simulink model "Simulink_drone_BO_facultatif"  (R2025b)
settings: Solver=VariableStepAuto  StartTime=0.0  StopTime=60  RelTol=1e-3
undefined symbols (not defined in the file): bool, controller, dt_realtime, sysBO, x_init
libraries: aerolibanimutils x2, uavsim3dlib x1, sim3dlib x1
settings Model: Creator=guilb  LastModifiedBy=guilb

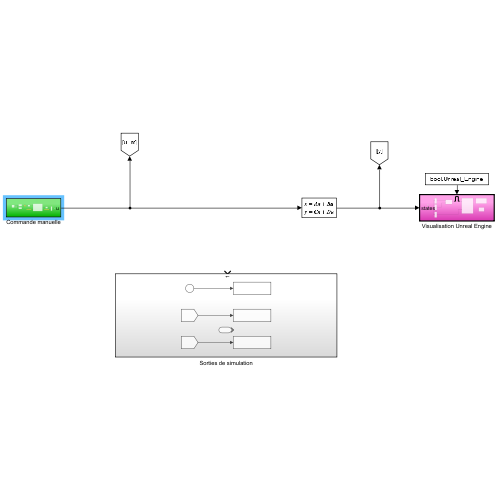
[thumbnail: Simulink's stored preview of the top-level diagram]
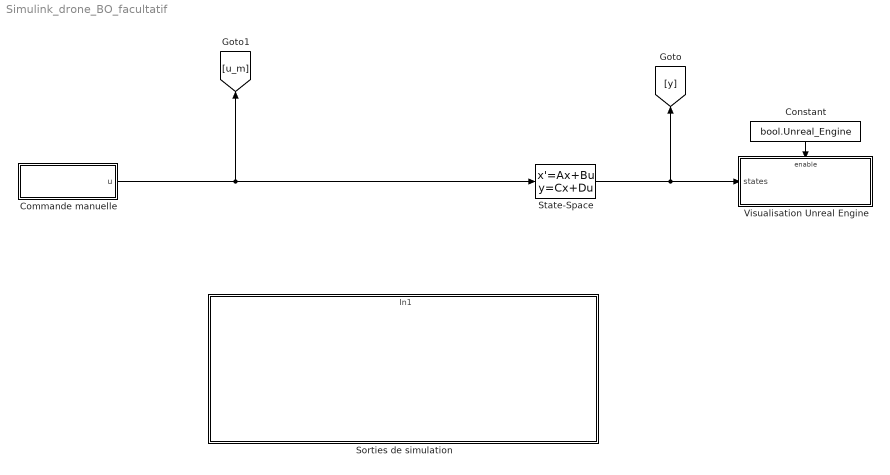
== system Simulink_drone_BO_facultatif ==
  Commande manuelle : Subsystem
  Constant : Constant  Value=bool.Unreal_Engine
  Sorties de simulation : Subsystem
      settings: PortSchema="{\"entries\":[{\"content\":{\"sides\":[{\"content\":{},\"type\":\"ConnectorPlacement.EquallySpacedRectSide\",\"uuid\":\"13ffba7f-bf1d-45b8-ba16-d739f7cf7d65\"},{\"content\":{\"side\":\"RIGHT\"},\"type\":\"ConnectorPlacement.EquallySpacedRectSide\",\"uuid\":\"a06d5891-851d-4d6f-ac4a-718ff50ccabc\"},{\"content\":{\"connectorIds\":[\"In1\"],\"side\":\"TOP\"},\"type\":\"ConnectorPlacement.EquallySpacedRectSide\",\"uuid\":\"896d5570-b42a-4582-b469-16ee5988ede6\"}]},\"type\":\"ConnectorPlacement.EquallySpacedConnector\",\"uuid\":\"8422d13c-e10a-49e8-a54f-6123e5432cb6\"}],\"packageUris\":[\"http://schema.mathworks.com/mf0/Connector/R2020b\"],\"version\":\"1.0\"}"
  State-Space : StateSpace  A=sysBO.A  B=sysBO.B  C=sysBO.C  D=sysBO.D  InitialCondition=x_init
  Visualisation Unreal Engine : Subsystem
  wires:
  Constant/1 -> Visualisation Unreal Engine/Enable
  State-Space/1 -> Visualisation Unreal Engine/1(states), [y]
  Commande manuelle/1(u) -> State-Space/1, [u_m]

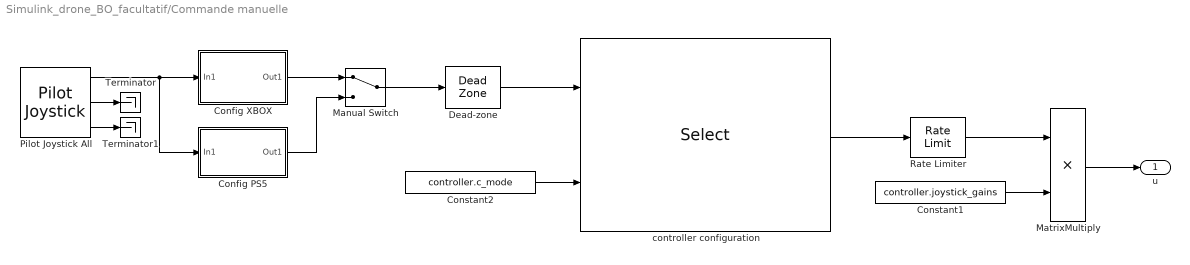
== system Simulink_drone_BO_facultatif/Commande manuelle ==
  Config PS5 : Subsystem
      mask Display: image('controller_ps5.png', [2,2,2,2,100,100]);
  "Config XBOX " : Subsystem
      mask Display: image('controller_xbox.png', [2,2,2,2,100,100]);
  Constant1 : Constant  Value=controller.joystick_gains
  Constant2 : Constant  Value=controller.c_mode
  Dead-zone : DeadZone  LowerValue=-0.2  UpperValue=0.2
  Manual Switch : ManualSwitch
  MatrixMultiply : Product
  Pilot Joystick All : aerolibanimutils/Pilot Joystick  JoystickID=Joystick1  OutputConfiguration=AllOutputs  SampleTime=dt_realtime
      settings: LibrarySourceBlock=aerolibanimutils/Pilot Joystick All
  "Rate Limiter " : RateLimiter  RisingSlewLimit=controller.rate_limits  FallingSlewLimit=-controller.rate_limits
  Terminator : Terminator
  Terminator1 : Terminator
  controller configuration : Selector  InputPortWidth=4  IndexOptions=Index vector (port)  Indices=[2 4 3 1]  OutputSizes=1
      mask Display: image('controller_modes.png');
  u : Outport
  wires:
  controller configuration/1 -> "Rate Limiter "/1
  MatrixMultiply/1 -> u/1
  Constant1/1 -> MatrixMultiply/2
  Constant2/1 -> controller configuration/2
  "Rate Limiter "/1 -> MatrixMultiply/1
  Dead-zone/1 -> controller configuration/1
  Pilot Joystick All/1 -> "Config XBOX "/1(In1), Config PS5/1(In1)
  Manual Switch/1 -> Dead-zone/1
  "Config XBOX "/1(Out1) -> Manual Switch/1
  Config PS5/1(Out1) -> Manual Switch/2
  Pilot Joystick All/2 -> Terminator/1
  Pilot Joystick All/3 -> Terminator1/1

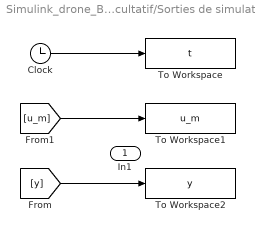
== system Simulink_drone_BO_facultatif/Sorties de simulation ==
  In1 : Inport
  Clock : Clock
  To Workspace : ToWorkspace  VariableName=t  SaveFormat=Timeseries  SampleTime=-1
  To Workspace1 : ToWorkspace  VariableName=u_m  SaveFormat=Timeseries  SampleTime=-1
  To Workspace2 : ToWorkspace  VariableName=y  SaveFormat=Timeseries  SampleTime=-1
  wires:
  Clock/1 -> To Workspace/1
  [y] -> To Workspace2/1
  [u_m] -> To Workspace1/1

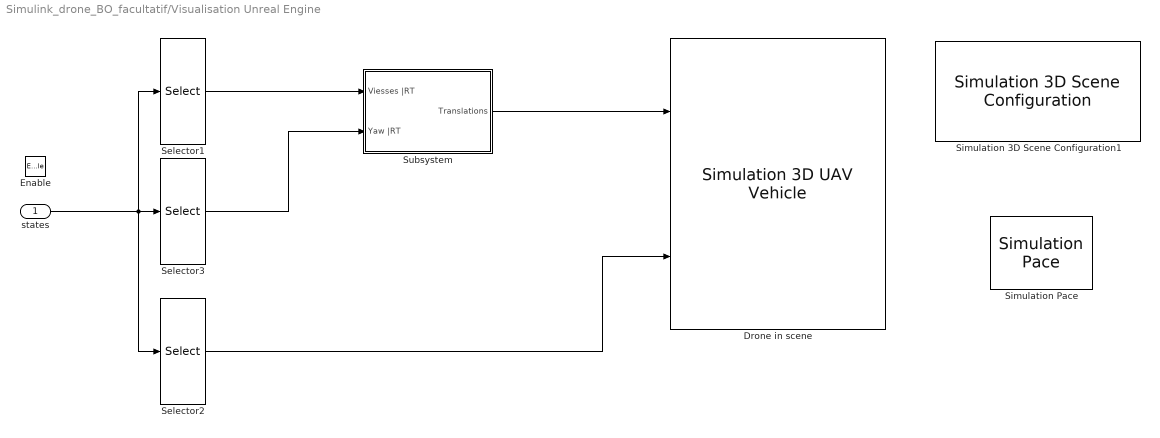
== system Simulink_drone_BO_facultatif/Visualisation Unreal Engine ==
  states : Inport
  Enable : EnablePort
  Drone in scene : uavsim3dlib/Simulation 3D UAV Vehicle  Priority=-1  Mesh=Quadrotor  MeshPath=/MathWorksUAVContent/UAVs/HexaRotorUAV/HexaRotor.HexaRotor  Color=Black  ActorName=SimulinkVehicle1  UseGlobalFrame=off  InitialTranslation=[0 0 0]  InitialRotation=[0 0 0]  InitialTranslationGlobal=[0 0 0]  InitialGeoOrigin=[0 0 0]  InitialRotationGlobal=[0 0 0]  SampleTime=-1  ActorType=SimulinkVehicle  ID=1  aMode=4  ActorTag=SimulinkVehicle1
  Selector1 : Selector  InputPortWidth=12  IndexOptions=Index vector (dialog)  Indices=[2 4 6]  OutputSizes=1
  Selector2 : Selector  InputPortWidth=12  IndexOptions=Index vector (dialog)  Indices=[11 9 7]  OutputSizes=1
  Selector3 : Selector  InputPortWidth=12  IndexOptions=Index vector (dialog)  Indices=11  OutputSizes=1
  Simulation 3D Scene Configuration1 : sim3dlib/Simulation 3D Scene Configuration  Priority=0  ProjectFormat=Default Scenes  SceneDesc=US city block  ProjectName=C:\Program Files\MATLAB\R2025b\toolbox\shared\sim3d_projects\automotive_project_windows\UE\WindowsNoEditor\VehicleSimulation.exe  ScenePath=/Game/Maps/USCityBlock  EnableOpenDRIVE=off  vehTagList={'Custom';'Scene Origin';'SimulinkVehicle1'}  vehTag=SimulinkVehicle1  AttachedCameraRelativeTranslation=[0 0 0]  FreeCameraDefaultInitialTranslation=[-6, 0, 2]  AttachedCameraRelativeRotation=[0 0 0]  FreeCameraDefaultInitialRotation=[0, -15, 0]  ViewpointName=Custom  FreeCameraInitialTranslation=[0, 0, 0]  ViewpointTranslation=[0 0 0]  FreeCameraInitialRotation=[0, 0, 0]  ViewpointRotation=[0 0 0]  OpVisEn=off  Ts=dt_realtime  EnableWindow=on  EnableRemoteAccess=off  EnableWeather=off  SunAzimuth=90  SunAltitude=40.0  EnableGeospatialSun=off  Latitude=0  Longitude=0  Date=2023-01-01  Time=10:30:00  GeoTimeZone=-5.0  SunDaylightSaving=off  wind=1  clouds=10  EnableVolumetricClouds=off  CloudCoverage=0  CloudAltitude=6  fog=0  rain=0  RaindropsEffect=off  SnowDensity=0  EnableGeospatial=off  TilesetSource=Earth terrain  UseTrueOrigin=off  OriginHeight=200  OriginLatitude=40.744652  OriginLongitude=-73.988864  MapStyle=Aerial  AdditionalAssetIDs=[]  UseAdvancedSunSky=off  SolarTime=11  TimeZone=-5  Day=21  Month=9  Year=2022  UseDaylightSavingTime=on  DSTStartDay=10  DSTStartMonth=3  DSTEndDay=3  DSTEndMonth=11  DSTSwitchHour=2  sensorTag=MainCamera1  sensorId=1  sensorName=MainCamera1  mountLoc=Origin  offsetFlag=off  tmountOffset=[0, 0, 0]  rmountOffset=[0, 0, 0]  HorizontalResolution=1280  VerticalResolution=720  HorizontalFOV=60  mountPoint=[0 0 0]  mountOrientation=[0 0 0]  aMode=4  ID=1  GeoTrigger=Inactive  ViewNameList={'Custom'}  ViewTranslationList={'[0 0 0]'}  ViewRotationList={'[0 0 0]'}
      settings: LibrarySourceBlock=uavsim3dlib/Simulation 3D Scene Configuration
  Simulation Pace : aerolibanimutils/Simulation Pace  SimulationPace=1  SleepMode=Auto  OutputPaceError=off  SampleTime=dt_realtime
  Subsystem : Subsystem
  wires:
  states/1 -> Selector1/1, Selector2/1, Selector3/1
  Selector2/1 -> Drone in scene/2
  Selector1/1 -> Subsystem/1(Viesses |RT)
  Selector3/1 -> Subsystem/2("Yaw |RT ")
  Subsystem/1(Translations) -> Drone in scene/1

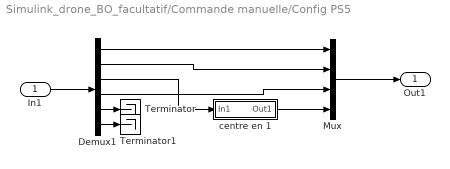
== system Simulink_drone_BO_facultatif/Commande manuelle/Config PS5 ==
  In1 : Inport
  Demux1 : Demux  Outputs=6
  Mux : Mux
  Terminator : Terminator
  Terminator1 : Terminator
  centre en 1 : Subsystem
  Out1 : Outport
  wires:
  Demux1/6 -> Terminator1/1
  Demux1/5 -> Terminator/1
  Demux1/4 -> Mux/3
  In1/1 -> Demux1/1
  Demux1/1 -> Mux/1
  Demux1/2 -> Mux/2
  Mux/1 -> Out1/1
  centre en 1/1(Out1) -> Mux/4
  Demux1/3 -> centre en 1/1(In1)

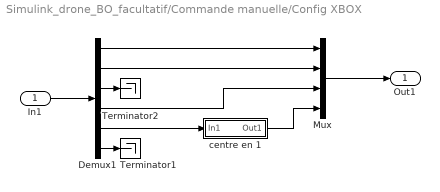
== system Simulink_drone_BO_facultatif/Commande manuelle/Config XBOX  ==
  In1 : Inport
  Demux1 : Demux  Outputs=6
  Mux : Mux
  Terminator1 : Terminator
  Terminator2 : Terminator
  centre en 1 : Subsystem
  Out1 : Outport
  wires:
  Mux/1 -> Out1/1
  Demux1/2 -> Mux/2
  Demux1/1 -> Mux/1
  In1/1 -> Demux1/1
  Demux1/6 -> Terminator1/1
  Demux1/4 -> Mux/3
  centre en 1/1(Out1) -> Mux/4
  Demux1/5 -> centre en 1/1(In1)
  Demux1/3 -> Terminator2/1

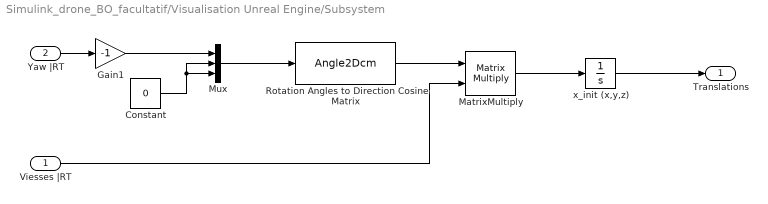
== system Simulink_drone_BO_facultatif/Visualisation Unreal Engine/Subsystem ==
  Viesses |RT : Inport
  "Yaw |RT " : Inport  Port=2
  Constant : Constant  Value=0
  Gain1 : Gain  Gain=-1
  MatrixMultiply : Product  Multiplication=Matrix(*)
  Mux : Mux  Inputs=3
  Rotation Angles to Direction Cosine Matrix : Angle2Dcm
      settings: AttributesFormatString=Rotation Order: %<rotationOrder>
  x_init (x,y,z) : Integrator  InitialCondition=[x_init(1) ; x_init(3) ; x_init(5)]
  Translations : Outport
  wires:
  Constant/1 -> Mux/2, Mux/3
  x_init (x,y,z)/1 -> Translations/1
  MatrixMultiply/1 -> x_init (x,y,z)/1
  Mux/1 -> Rotation Angles to Direction Cosine Matrix/1
  Rotation Angles to Direction Cosine Matrix/1 -> MatrixMultiply/1
  "Yaw |RT "/1 -> Gain1/1
  Viesses |RT/1 -> MatrixMultiply/2
  Gain1/1 -> Mux/1

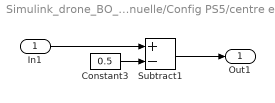
== system Simulink_drone_BO_facultatif/Commande manuelle/Config PS5/centre en 1 ==
  In1 : Inport
  Constant3 : Constant  Value=0.5
  Subtract1 : Sum  Inputs=+-
  Out1 : Outport
  wires:
  Subtract1/1 -> Out1/1
  In1/1 -> Subtract1/1
  Constant3/1 -> Subtract1/2

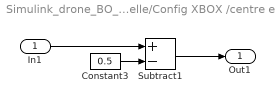
== system Simulink_drone_BO_facultatif/Commande manuelle/Config XBOX /centre en 1 ==
  In1 : Inport
  Constant3 : Constant  Value=0.5
  Subtract1 : Sum  Inputs=+-
  Out1 : Outport
  wires:
  Subtract1/1 -> Out1/1
  In1/1 -> Subtract1/1
  Constant3/1 -> Subtract1/2
